simulink model "Lab_0"  (R2025b)
settings: Solver=ode1  StartTime=0.0  StopTime=15.0  FixedStep=.01  RelTol=1e-3
settings Model: Creator=ASUS  LastModifiedBy=ASUS

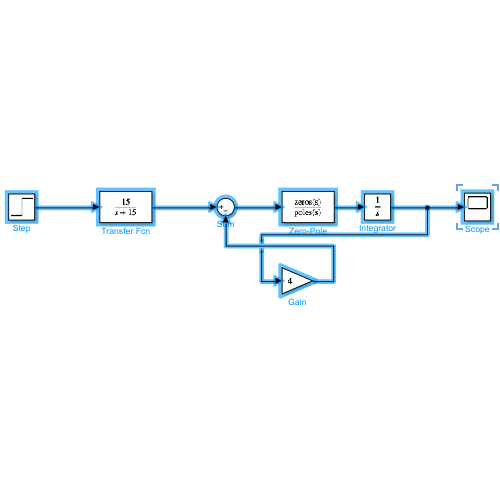
[thumbnail: Simulink's stored preview of the top-level diagram]
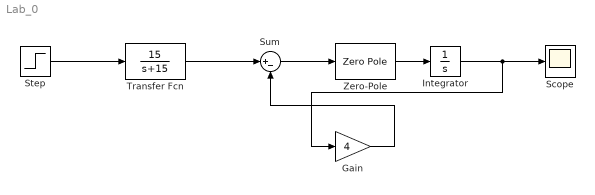
== system Lab_0 ==
  Gain : Gain  Gain=4
  Integrator : Integrator
  Scope : Scope
  Step : Step  Time=2  Before=1  After=4  SampleTime=0
  Sum : Sum  Inputs=|+-
  Transfer Fcn : TransferFcn  Numerator=15  Denominator=[1 15]
  Zero-Pole : ZeroPole  Zeros=[1 10]  Poles=[1 1]
  wires:
  Step/1 -> Transfer Fcn/1
  Transfer Fcn/1 -> Sum/1
  Sum/1 -> Zero-Pole/1
  Zero-Pole/1 -> Integrator/1
  Integrator/1 -> Gain/1, Scope/1
  Gain/1 -> Sum/2
